simulink model "ARI_20_3_AW_4_5"  (Simulink 7.8)
settings: Solver=ode45  StartTime=0.0  StopTime=10.0  RelTol=1e-3
values from neighbouring files (symbols this model uses):
  h = findobj(gcf,'type','line')    [boldLines.m]    (also in phase.m = min(hmax, 0.9*h*(tau/delta)^pow))
undefined symbols (not defined in the file or in its folder): A, B, C, D
settings Model: Creator=Michael Sebek  ModifiedByFormat=Michael Sebek  LastModifiedBy=Michael Sebek
settings OptimizationCC: InitFltsAndDblsToZero=on
settings DebuggingCC: SaveWithParameterizedLinksMsg=none  SignalResolutionControl=TryResolveAllWithWarning  MultiTaskDSMMsg=warning  MultiTaskCondExecSysMsg=none  FcnCallInpInsideContextMsg=Use local settings  StrictBusMsg=None
settings RTWCC: IncludeERTFirstTime=on
settings GRTTargetCC: TargetFcnLib=ansi_tfl_tmw.mat

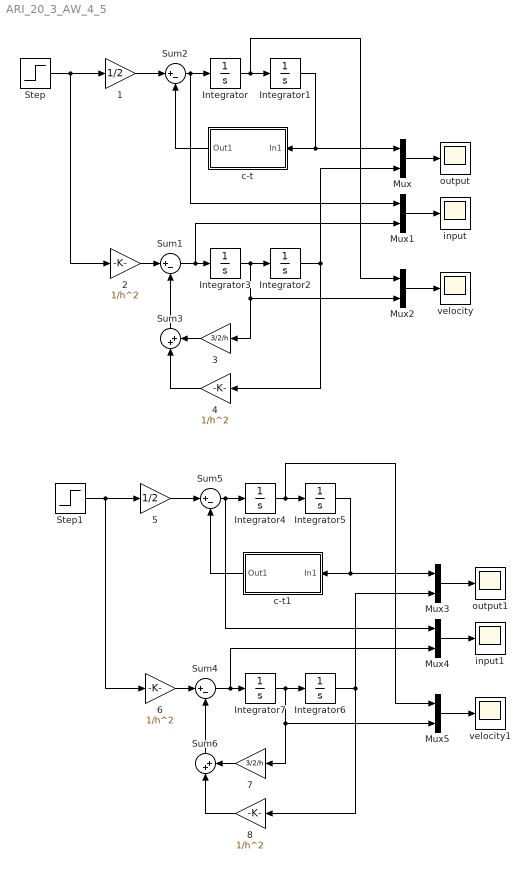
== system ARI_20_3_AW_4_5 ==
  1 : Gain  Gain=1/2
  2 : Gain  Gain=1/h^2
  3 : Gain  Gain=3/2/h  SampleTime=h
  4 : Gain  Gain=1/h^2  SampleTime=h
  5 : Gain  Gain=1/2
  6 : Gain  Gain=1/h^2
  7 : Gain  Gain=3/2/h  SampleTime=h
  8 : Gain  Gain=1/h^2  SampleTime=h
  Integrator{,1..3} (4 alike) : Integrator
  Integrator4 : Integrator  InitialCondition=2
  Integrator5 : Integrator  InitialCondition=-1
  Integrator6 : Integrator  InitialCondition=-1
  Integrator7 : Integrator  InitialCondition=2
  Mux{,1..5} (6 alike) : Mux  Inputs=2
  Step : Step  Time=0  SampleTime=0
  Step1 : Step  Time=0  SampleTime=0
  Sum{1..2,4..5} (4 alike) : Sum  Inputs=|+-
  Sum3 : Sum  Inputs=|++
  Sum6 : Sum  Inputs=|++
  c-t : Subsystem  mask(PMF Block){F=2*(s+.5)/(s+2), InCon=[ ], SampTime=1, fvar=No change}
      mask prompts: F "PMF Object:"; InCon "Initial states:"; SampTime "Sample time (discrete time only):"; fvar "Force variable:"
      mask help:
      | Polynomial matrix fraction description of a linear system.
      |
      | This block represents a linear system defined by the polynomial matrix fraction of its transfer function.
      mask init:
      | Label = 'xxx';
      | [A,B,C,D,Label,var] = polymask2(F, fvar, length(InCon));
      | update;
      mask Help:
      | This block represents a linear system [<I>A,B,C,D</I>] defined by the polynomial matrix fraction (<I>PMF</I>) of its transfer function <I>T</I>.
      | <p>
      | <b>Left Matrix Fraction</b> item of the popup menu <b>Type</b> indicates the transfer function in the form of <I>left PMF</I>:
      | <p>
      | <I>T</I> = inv(<I>Q</I>) <I>P</I>.
      | <p>
      | <b>Right Matrix Fraction</b> item is used if the transfer function is given in the form of <I>right PMF</I>:
      | <p>
      | <I>T</I> = <I>P</I> inv(<I>Q</I>).
      | <p>
      |  The <b>variable</b> determines the type  of the system:
      | <p>
      | - <b>s, p</b> are used for continous time systems (Laplace transform).
      | <p>
      | - <b>z, q</b> are used for discrete time transfer functions in forward-shift operator (Z-transform).
      | <p>
      | - <b>d, z^-1</b> are used for discrete time transfer functions in backward-shift operator.
      | <p>
      | <b> Note:</b> For the variables <I>s,p,z,q</I>, the transfer function is defined as
      | <p>
      | <I>T</I> = <I>C</I> inv(<I>vI-A</I>) <I>B</I> + <I>D</I>,
      | <p>
      | where <I>v</I> is the variable of <I>P,Q</I>.
      | For the variables <I>d, z^-1</I>, the transfer function is defined as
      | <p>
      | <I>T</I> = <I>C v</I> inv(<I>I-Av</I>)  <I>B</I> + <I>D</I>.
      | <p>
      | <b>Note:</b> <b>Initial states</b> concern the observer-form realization of the system as defined by LMF2S and RMF2S functions. Their number must equal the sum of column degrees of the denominator matrix <I>Q</I> in case of right PMF and the sum of row degrees of <I>Q</I> for left PMF description.
      | <p>
      | See also POL, LMF2S, RMF2S.
      mask StyleString: edit,edit,edit,popup(No change|s   (continous time)|p   (continous time)|z      (discrete time)|q      (discrete time)|d      (discrete time)|z^-1 (discrete time))
      mask Display: droots([-.5], [-2], 2)
  c-t1 : Subsystem  mask(PMF Block){F=2*(s+.5)/(s+2), InCon=[ ], SampTime=1, fvar=No change}
      mask prompts: F "PMF Object:"; InCon "Initial states:"; SampTime "Sample time (discrete time only):"; fvar "Force variable:"
      mask help:
      | Polynomial matrix fraction description of a linear system.
      |
      | This block represents a linear system defined by the polynomial matrix fraction of its transfer function.
      mask init:
      | Label = 'xxx';
      | [A,B,C,D,Label,var] = polymask2(F, fvar, length(InCon));
      | update;
      mask Help:
      | This block represents a linear system [<I>A,B,C,D</I>] defined by the polynomial matrix fraction (<I>PMF</I>) of its transfer function <I>T</I>.
      | <p>
      | <b>Left Matrix Fraction</b> item of the popup menu <b>Type</b> indicates the transfer function in the form of <I>left PMF</I>:
      | <p>
      | <I>T</I> = inv(<I>Q</I>) <I>P</I>.
      | <p>
      | <b>Right Matrix Fraction</b> item is used if the transfer function is given in the form of <I>right PMF</I>:
      | <p>
      | <I>T</I> = <I>P</I> inv(<I>Q</I>).
      | <p>
      |  The <b>variable</b> determines the type  of the system:
      | <p>
      | - <b>s, p</b> are used for continous time systems (Laplace transform).
      | <p>
      | - <b>z, q</b> are used for discrete time transfer functions in forward-shift operator (Z-transform).
      | <p>
      | - <b>d, z^-1</b> are used for discrete time transfer functions in backward-shift operator.
      | <p>
      | <b> Note:</b> For the variables <I>s,p,z,q</I>, the transfer function is defined as
      | <p>
      | <I>T</I> = <I>C</I> inv(<I>vI-A</I>) <I>B</I> + <I>D</I>,
      | <p>
      | where <I>v</I> is the variable of <I>P,Q</I>.
      | For the variables <I>d, z^-1</I>, the transfer function is defined as
      | <p>
      | <I>T</I> = <I>C v</I> inv(<I>I-Av</I>)  <I>B</I> + <I>D</I>.
      | <p>
      | <b>Note:</b> <b>Initial states</b> concern the observer-form realization of the system as defined by LMF2S and RMF2S functions. Their number must equal the sum of column degrees of the denominator matrix <I>Q</I> in case of right PMF and the sum of row degrees of <I>Q</I> for left PMF description.
      | <p>
      | See also POL, LMF2S, RMF2S.
      mask StyleString: edit,edit,edit,popup(No change|s   (continous time)|p   (continous time)|z      (discrete time)|q      (discrete time)|d      (discrete time)|z^-1 (discrete time))
      mask Display: droots([-.5], [-2], 2)
  input : Scope
      settings: SaveName=ScopeData2
  input1 : Scope
  output : Scope
      settings: SaveName=ScopeData3
  output1 : Scope
      settings: SaveName=ScopeData4
  velocity : Scope
  velocity1 : Scope
      settings: SaveName=ScopeData5
  wires:
  Integrator1/1 -> c-t/1(In1), Mux/1
  Sum2/1 -> Mux1/1, Integrator/1
  1/1 -> Sum2/1
  Step/1 -> 1/1, 2/1
  c-t/1(Out1) -> Sum2/2
  Integrator2/1 -> Mux/2, 4/1
  Sum1/1 -> Mux1/2, Integrator3/1
  2/1 -> Sum1/1
  Mux/1 -> output/1
  Mux1/1 -> input/1
  Integrator/1 -> Integrator1/1, Mux2/1
  Integrator3/1 -> Integrator2/1, Mux2/2, 3/1
  Mux2/1 -> velocity/1
  Sum3/1 -> Sum1/2
  4/1 -> Sum3/1
  3/1 -> Sum3/2
  Integrator5/1 -> Mux3/1, c-t1/1(In1)
  Sum5/1 -> Integrator4/1, Mux4/1
  5/1 -> Sum5/1
  Step1/1 -> 6/1, 5/1
  c-t1/1(Out1) -> Sum5/2
  Integrator6/1 -> 8/1, Mux3/2
  Sum4/1 -> Integrator7/1, Mux4/2
  6/1 -> Sum4/1
  Mux3/1 -> output1/1
  Mux4/1 -> input1/1
  Integrator4/1 -> Mux5/1, Integrator5/1
  Integrator7/1 -> 7/1, Mux5/2, Integrator6/1
  Mux5/1 -> velocity1/1
  Sum6/1 -> Sum4/2
  8/1 -> Sum6/1
  7/1 -> Sum6/2

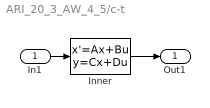
== system ARI_20_3_AW_4_5/c-t ==
  In1 : Inport
  Inner : StateSpace  A=A  B=B  C=C  D=D  X0=InCon
  Out1 : Outport
  wires:
  In1/1 -> Inner/1
  Inner/1 -> Out1/1

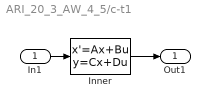
== system ARI_20_3_AW_4_5/c-t1 ==
  In1 : Inport
  Inner : StateSpace  A=A  B=B  C=C  D=D  X0=InCon
  Out1 : Outport
  wires:
  Inner/1 -> Out1/1
  In1/1 -> Inner/1
